simulink model "SMM_1_roughT"  (Simulink 8.1)
settings: Solver=ode45  StartTime=0.0  StopTime=20  MaxStep=1e-3  RelTol=1e-4  AbsTol=1e-6
values from neighbouring files (symbols this model uses):
  alpha0 = 68  *pi/180    (= 1.18682389136)    [SMM_1_params.m]    (also in SMM_1_returnMap.m; SMM_1_roughTerrain.m)
  dx0 = 5    [SMM_1_params.m]    (also in SMM_1_returnMap.m = sqrt(2/m*(Esys-m*g*y0)))
  dy0 = 0    [SMM_1_params.m]    (also in SMM_1_returnMap.m; SMM_1_roughTerrain.m)
  g = 9.81    [SMM_1_params.m]    (also in SMM_1_returnMap.m; SMM_1_roughTerrain.m)
  Grndmax = 0.01    [SMM_1_params.m]    (also in SMM_1_roughTerrain.m = 0.15)
  k = 20000    [SMM_1_params.m]    (also in SMM_1_returnMap.m; SMM_1_roughTerrain.m)
  l0 = 1    [SMM_1_params.m]    (also in SMM_1_returnMap.m; SMM_1_roughTerrain.m)
  m = 70    [SMM_1_params.m]    (also in SMM_1_returnMap.m; SMM_1_roughTerrain.m)
  x0 = 0    [SMM_1_params.m]    (also in SMM_1_returnMap.m; SMM_1_roughTerrain.m)
  y0 = 1    [SMM_1_params.m]    (also in SMM_1_returnMap.m = v_y0(state))
libraries: simulink_extras x1
settings Model: Creator=hgeyer  LastModifiedBy=benshih
settings DebuggingCC: FcnCallInpInsideContextMsg=EnableAllAsWarning
settings GRTTargetCC: CombineOutputUpdateFcns=on  GRTInterface=off

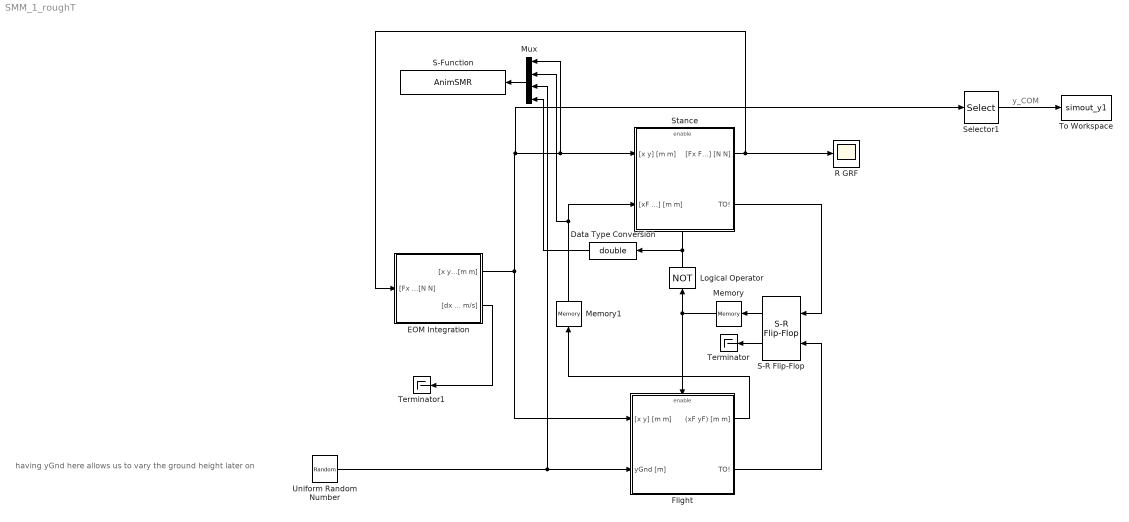
== system SMM_1_roughT ==
  note: y_COM
  note: having yGnd here allows
      | us to vary the ground height later on
  Data Type Conversion : DataTypeConversion  OutDataTypeStr=double
  EOM Integration : Subsystem
  Flight : Subsystem
  Logical Operator : Logic  Operator=NOT  AllPortsSameDT=off  OutDataTypeStr=boolean
  Memory : Memory  X0=1
  Memory1 : Memory  X0=[0 0]
  Mux : Mux
  R GRF : Scope
  S-Function : S-Function  FunctionName=AnimSMR  Parameters=0.01  EnableBusSupport=off
  S-R Flip-Flop : simulink_extras/Flip Flops/S-R Flip-Flop  initial_condition=1
  Selector1 : Selector  InputPortWidth=2  IndexOptions=Index vector (dialog)  Indices=2  OutputSizes=1
  Stance : Subsystem
  Terminator : Terminator
  Terminator1 : Terminator
  To Workspace : ToWorkspace  VariableName=simout_y1  SampleTime=-1
      settings: MaxDataPoints=1
  Uniform Random Number : UniformRandomNumber  Minimum=-Grndmax/2  Maximum=Grndmax/2  SampleTime=0.1
  wires:
  EOM Integration/1("[x y] [m m]") -> Flight/1("[x y] [m m]"), Selector1/1, Mux/1, Stance/1("[x y] [m m]")
  Stance/2(TO!) -> S-R Flip-Flop/1
  S-R Flip-Flop/1 -> Memory/1
  Logical Operator/1 -> Stance/Enable, Data Type Conversion/1
  Memory/1 -> Logical Operator/1, Flight/Enable
  Flight/2(TO!) -> S-R Flip-Flop/2
  Flight/1((xF yF) [m m]) -> Memory1/1
  Memory1/1 -> Mux/2, Stance/2("[xF yF] [m m]")
  Mux/1 -> S-Function/1
  S-R Flip-Flop/2 -> Terminator/1
  Stance/1("[Fx Fy] [N N]") -> R GRF/1, EOM Integration/1("[Fx Fy] [N N]")
  Uniform Random Number/1 -> Flight/2(yGnd [m]), Mux/3
  Data Type Conversion/1 -> Mux/4
  Selector1/1 -> To Workspace/1
  EOM Integration/2("[dx dy] [m/s m/s]") -> Terminator1/1

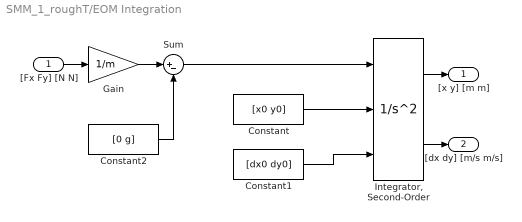
== system SMM_1_roughT/EOM Integration ==
  "[Fx Fy] [N N]" : Inport
  Constant : Constant  Value=[x0 y0]
  Constant1 : Constant  Value=[dx0 dy0]
  Constant2 : Constant  Value=[0 g]
  Gain : Gain  Gain=1/m
  "Integrator, Second-Order" : SecondOrderIntegrator  ICSourceX=external  ICSourceDXDT=external
  Sum : Sum  Inputs=|+-
  "[x y] [m m]" : Outport
  "[dx dy] [m/s m/s]" : Outport  Port=2
  wires:
  Constant/1 -> "Integrator, Second-Order"/2
  Constant1/1 -> "Integrator, Second-Order"/3
  Gain/1 -> Sum/1
  Sum/1 -> "Integrator, Second-Order"/1
  Constant2/1 -> Sum/2
  "[Fx Fy] [N N]"/1 -> Gain/1
  "Integrator, Second-Order"/1 -> "[x y] [m m]"/1
  "Integrator, Second-Order"/2 -> "[dx dy] [m/s m/s]"/1

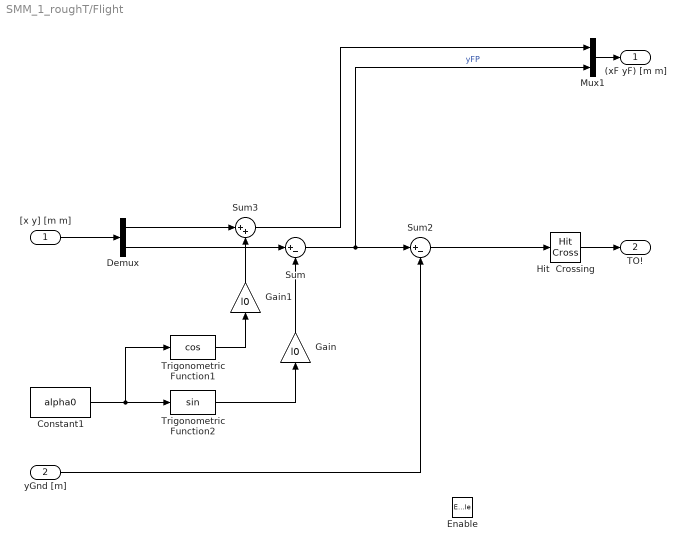
== system SMM_1_roughT/Flight ==
  "[x y] [m m]" : Inport
  yGnd [m] : Inport  Port=2
  Enable : EnablePort  StatesWhenEnabling=reset
  Constant1 : Constant  Value=alpha0
  Demux : Demux  Outputs=2
  Gain : Gain  Gain=l0
  Gain1 : Gain  Gain=l0
  Hit  Crossing : HitCross  HitCrossingDirection=falling
  Mux1 : Mux  Inputs=2
  Sum : Sum  Inputs=|+-
  Sum2 : Sum  Inputs=|+-
  Sum3 : Sum  Inputs=|++
  Trigonometric Function1 : Trigonometry  Operator=cos
  Trigonometric Function2 : Trigonometry
  (xF yF) [m m] : Outport  InitialOutput=0
  TO! : Outport  Port=2  OutputWhenDisabled=reset  InitialOutput=0
  wires:
  Hit  Crossing/1 -> TO!/1
  Mux1/1 -> (xF yF) [m m]/1
  "[x y] [m m]"/1 -> Demux/1
  Demux/2 -> Sum/1
  Constant1/1 -> Trigonometric Function2/1, Trigonometric Function1/1
  Trigonometric Function2/1 -> Gain/1
  Gain/1 -> Sum/2
  Sum/1 -> Sum2/1, Mux1/2  "yFP"
  yGnd [m]/1 -> Sum2/2
  Sum2/1 -> Hit  Crossing/1
  Trigonometric Function1/1 -> Gain1/1
  Gain1/1 -> Sum3/2
  Demux/1 -> Sum3/1
  Sum3/1 -> Mux1/1

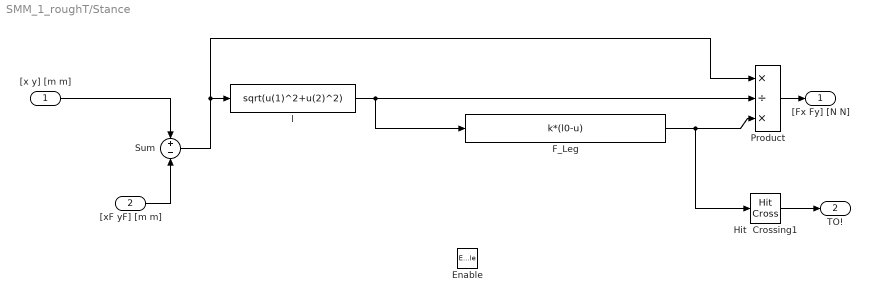
== system SMM_1_roughT/Stance ==
  "[x y] [m m]" : Inport
  "[xF yF] [m m]" : Inport  Port=2
  Enable : EnablePort  StatesWhenEnabling=reset
  F_Leg : Fcn  Expr=k*(l0-u)
  Hit  Crossing1 : HitCross  HitCrossingDirection=falling
  Product : Product  Inputs=*/*  RndMeth=Zero
  Sum : Sum  Inputs=+-
  l : Fcn  Expr=sqrt(u(1)^2+u(2)^2)
  "[Fx Fy] [N N]" : Outport  OutputWhenDisabled=reset  InitialOutput=[0 0]
  TO! : Outport  Port=2  OutputWhenDisabled=reset  InitialOutput=0
  wires:
  F_Leg/1 -> Product/3, Hit  Crossing1/1
  l/1 -> Product/2, F_Leg/1
  Product/1 -> "[Fx Fy] [N N]"/1
  "[xF yF] [m m]"/1 -> Sum/2
  "[x y] [m m]"/1 -> Sum/1
  Sum/1 -> l/1, Product/1
  Hit  Crossing1/1 -> TO!/1
